simulink model "Kalmanfilter"  (R2021a)
settings: Solver=VariableStepAuto  StartTime=0.0  StopTime=10.0  RelTol=1e-3
undefined symbols (not defined in the file): A, B, C1
settings Model: Creator=shrutidalal  LastModifiedBy=shrutidalal

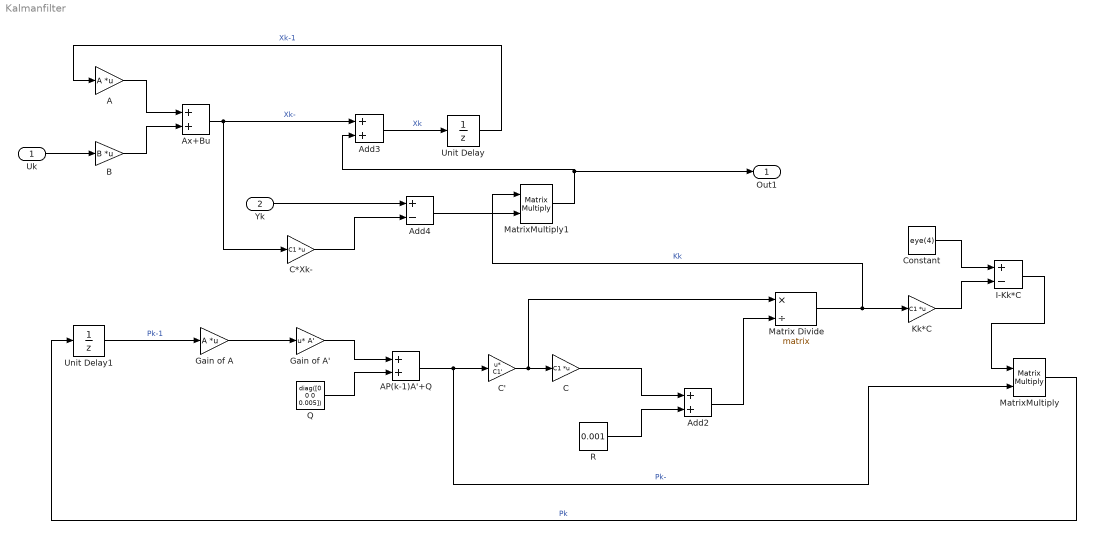
== system Kalmanfilter ==
  Uk : Inport
  Yk : Inport  Port=2
  A : Gain  Gain=A  Multiplication=Matrix(K*u)
  AP(k-1)A'+Q : Sum
  Add2 : Sum
  Add3 : Sum
  Add4 : Sum  Inputs=+-
  Ax+Bu : Sum
  B : Gain  Gain=B  Multiplication=Matrix(K*u)
  C : Gain  Gain=C1  Multiplication=Matrix(K*u)
  C' : Gain  Gain=C1'  Multiplication=Matrix(u*K)
  C*Xk- : Gain  Gain=C1  Multiplication=Matrix(K*u)
  Constant : Constant  Value=eye(4)
  Gain of A : Gain  Gain=A  Multiplication=Matrix(K*u)
  Gain of A' : Gain  Gain=A'  Multiplication=Matrix(u*K)
  I-Kk*C : Sum  Inputs=+-
  Kk*C : Gain  Gain=C1  Multiplication=Matrix(K*u)
  Matrix Divide : Product  Inputs=*/  Multiplication=Matrix(*)
  MatrixMultiply : Product  Multiplication=Matrix(*)
  MatrixMultiply1 : Product  Multiplication=Matrix(*)
  Q : Constant  Value=diag([0 0 0 0.005])
  R : Constant  Value=0.001
  Unit Delay : UnitDelay  SampleTime=-1  HasFrameUpgradeWarning=on
  Unit Delay1 : UnitDelay  SampleTime=-1  HasFrameUpgradeWarning=on
  Out1 : Outport
  wires:
  A/1 -> Ax+Bu/1
  Yk/1 -> Add4/1
  C/1 -> Add2/1
  C*Xk-/1 -> Add4/2
  B/1 -> Ax+Bu/2
  Q/1 -> AP(k-1)A'+Q/2
  Add4/1 -> MatrixMultiply1/2
  AP(k-1)A'+Q/1 -> MatrixMultiply/2, C'/1  "Pk-"
  C'/1 -> Matrix Divide/1, C/1
  Uk/1 -> B/1
  Ax+Bu/1 -> C*Xk-/1, Add3/1  "Xk-"
  MatrixMultiply/1 -> Unit Delay1/1  "Pk"
  MatrixMultiply1/1 -> Add3/2, Out1/1
  Gain of A/1 -> Gain of A'/1
  Constant/1 -> I-Kk*C/1
  Kk*C/1 -> I-Kk*C/2
  Unit Delay1/1 -> Gain of A/1  "Pk-1"
  Unit Delay/1 -> A/1  "Xk-1"
  Gain of A'/1 -> AP(k-1)A'+Q/1
  I-Kk*C/1 -> MatrixMultiply/1
  R/1 -> Add2/2
  Matrix Divide/1 -> MatrixMultiply1/1, Kk*C/1  "Kk"
  Add2/1 -> Matrix Divide/2
  Add3/1 -> Unit Delay/1  "Xk"
